simulink model "VACModel"  (Simulink 8.3)
settings: Solver=ode1  SolverMode=MultiTasking  StartTime=0.0  StopTime=24  FixedStep=Ts_base  MaxStep=Ts_base  MinStep=1e-6  RelTol=1e-6
PreLoadFcn:
  | initModel
StopFcn:
  | overview
undefined symbols (not defined in the file): automatic, controller_sampling_frequency, Fixed, gcr, MVs, PI, signal, transmitter_deadtime, transmitter_sampling_frequency, Ts_save, y_ss
libraries: VAlib x96
(part 1 of 18)
settings Model: Creator=pydipalli  LastModifiedBy=lexx
settings SolverCC: AutoInsertRateTranBlk=on
settings DataIOCC: LimitDataPoints=off  SignalLoggingSaveFormat=Dataset  SaveOutput=off  SignalLogging=off  DSMLogging=off  SaveTime=off  StateSaveName=xx  TimeSaveName=tt
settings OptimizationCC: ExpressionDepthLimit=2147483647  InitFltsAndDblsToZero=on
settings DebuggingCC: AlgebraicLoopMsg=none  SaveWithDisabledLinksMsg=none  SaveWithParameterizedLinksMsg=none  SignalResolutionControl=TryResolveAllWithWarning  SolverPrmCheckMsg=none  InheritedTsInSrcMsg=none  MultiTaskDSMMsg=warning  MultiTaskCondExecSysMsg=none  FcnCallInpInsideContextMsg=UseLocalSettings  UnconnectedInputMsg=none  UnconnectedOutputMsg=none
settings HardwareCC: TargetUnknown=on
settings RTWCC: IncludeERTFirstTime=on
settings GRTTargetCC: TargetFcnLib=ansi_tfl_tmw.mat

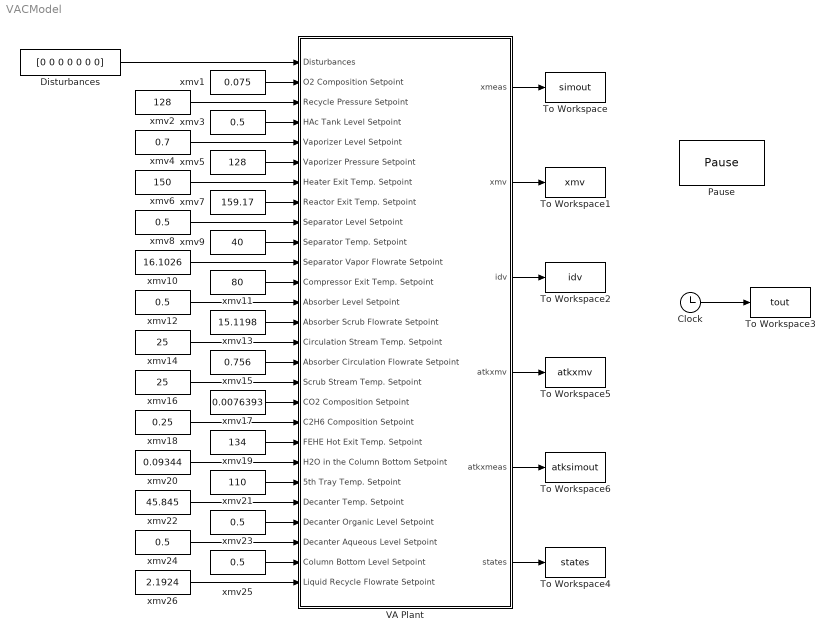
== system VACModel ==
  Clock : Clock
  Disturbances : Constant  Value=[0 0 0 0 0 0 0]
  Pause : VAlib/Pause  Value=-1
  To Workspace : ToWorkspace  VariableName=simout  SampleTime=Ts_save
  To Workspace1 : ToWorkspace  VariableName=xmv  SampleTime=Ts_save
  To Workspace2 : ToWorkspace  VariableName=idv  SampleTime=Ts_save
  To Workspace3 : ToWorkspace  VariableName=tout  SampleTime=Ts_save
      settings: Save2DSignal=2-D array (concatenate along first dimension)
  To Workspace4 : ToWorkspace  VariableName=states  SampleTime=Ts_save
  To Workspace5 : ToWorkspace  VariableName=atkxmv  SampleTime=Ts_save
  To Workspace6 : ToWorkspace  VariableName=atksimout  SampleTime=Ts_save
  VA Plant : Subsystem
  xmv1 : Constant  Value=0.075
  xmv10 : Constant  Value=16.1026
  xmv11 : Constant  Value=80
  xmv{3,8,12,23..25} (6 alike) : Constant  Value=0.5
  xmv13 : Constant  Value=15.1198
  xmv14 : Constant  Value=25
  xmv15 : Constant  Value=0.756
  xmv16 : Constant  Value=25
  xmv17 : Constant  Value=0.0076393
  xmv18 : Constant  Value=0.25
  xmv19 : Constant  Value=134
  xmv2 : Constant  Value=128
  xmv20 : Constant  Value=0.09344
  xmv21 : Constant  Value=110
  xmv22 : Constant  Value=45.845
  xmv26 : Constant  Value=2.1924
  xmv4 : Constant  Value=0.7
  xmv5 : Constant  Value=128
  xmv6 : Constant  Value=150
  xmv7 : Constant  Value=159.17
  xmv9 : Constant  Value=40
  wires:
  VA Plant/1(xmeas) -> To Workspace/1
  xmv2/1 -> VA Plant/3(Recycle Pressure Setpoint)
  VA Plant/2(xmv) -> To Workspace1/1
  VA Plant/3(idv) -> To Workspace2/1
  Clock/1 -> To Workspace3/1
  Disturbances/1 -> VA Plant/1(Disturbances)
  VA Plant/4(atkxmv) -> To Workspace5/1
  VA Plant/5(atkxmeas) -> To Workspace6/1
  xmv1/1 -> VA Plant/2(O2 Composition Setpoint)
  xmv3/1 -> VA Plant/4(HAc Tank Level Setpoint)
  xmv4/1 -> VA Plant/5(Vaporizer Level Setpoint)
  xmv5/1 -> VA Plant/6(Vaporizer Pressure Setpoint)
  xmv6/1 -> VA Plant/7(Heater Exit Temp. Setpoint)
  xmv7/1 -> VA Plant/8(Reactor Exit Temp. Setpoint)
  xmv8/1 -> VA Plant/9(Separator Level Setpoint)
  xmv9/1 -> VA Plant/10(Separator Temp. Setpoint)
  xmv10/1 -> VA Plant/11(Separator Vapor Flowrate Setpoint)
  xmv11/1 -> VA Plant/12(Compressor Exit Temp. Setpoint)
  xmv12/1 -> VA Plant/13(Absorber Level Setpoint)
  xmv13/1 -> VA Plant/14(Absorber Scrub Flowrate Setpoint)
  xmv14/1 -> VA Plant/15(Circulation Stream Temp. Setpoint)
  xmv15/1 -> VA Plant/16(Absorber Circulation Flowrate Setpoint)
  xmv16/1 -> VA Plant/17(Scrub Stream Temp. Setpoint)
  xmv17/1 -> VA Plant/18(CO2 Composition Setpoint)
  xmv18/1 -> VA Plant/19(C2H6 Composition Setpoint)
  xmv19/1 -> VA Plant/20(FEHE Hot Exit Temp. Setpoint)
  xmv20/1 -> VA Plant/21(H2O in the Column Bottom Setpoint)
  xmv21/1 -> VA Plant/22(5th Tray Temp. Setpoint)
  xmv22/1 -> VA Plant/23(Decanter Temp. Setpoint)
  xmv23/1 -> VA Plant/24(Decanter Organic Level Setpoint)
  xmv24/1 -> VA Plant/25(Decanter Aqueous Level Setpoint)
  xmv25/1 -> VA Plant/26(Column Bottom Level Setpoint)
  xmv26/1 -> VA Plant/27(Liquid Recycle Flowrate Setpoint)
  VA Plant/6(states) -> To Workspace4/1

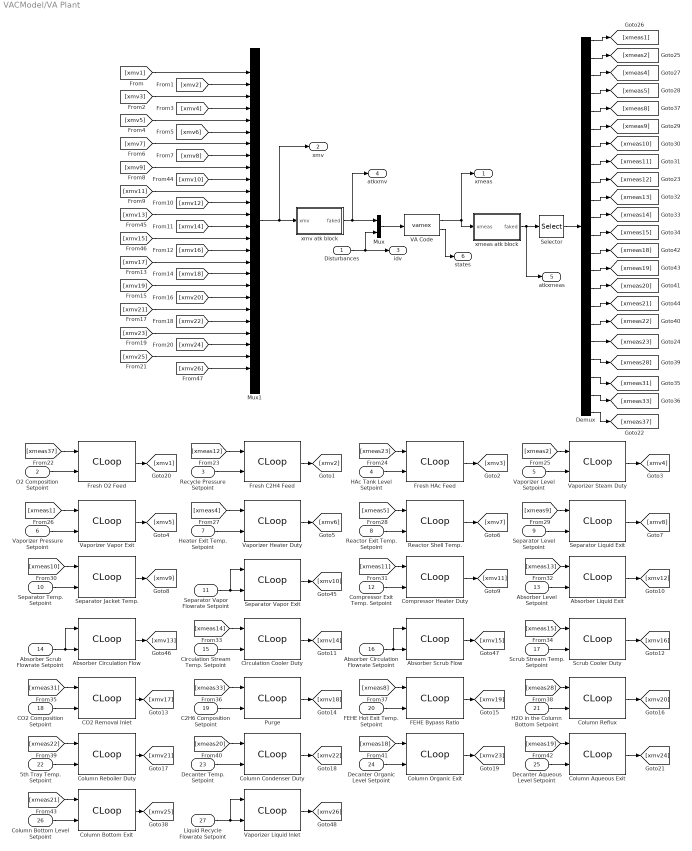
== system VACModel/VA Plant ==
  Disturbances : Inport
  O2 Composition Setpoint : Inport  Port=2
  Recycle Pressure Setpoint : Inport  Port=3
  HAc Tank Level Setpoint : Inport  Port=4
  Vaporizer Level Setpoint : Inport  Port=5
  Vaporizer Pressure Setpoint : Inport  Port=6
  Heater Exit Temp. Setpoint : Inport  Port=7
  Reactor Exit Temp. Setpoint : Inport  Port=8
  Separator Level Setpoint : Inport  Port=9
  Separator Temp. Setpoint : Inport  Port=10
  Separator Vapor Flowrate Setpoint : Inport  Port=11
  Compressor Exit Temp. Setpoint : Inport  Port=12
  Absorber Level Setpoint : Inport  Port=13
  Absorber Scrub Flowrate Setpoint : Inport  Port=14
  Circulation Stream Temp. Setpoint : Inport  Port=15
  Absorber Circulation Flowrate Setpoint : Inport  Port=16
  Scrub Stream Temp. Setpoint : Inport  Port=17
  CO2 Composition Setpoint : Inport  Port=18
  C2H6 Composition Setpoint : Inport  Port=19
  FEHE Hot Exit Temp. Setpoint : Inport  Port=20
  H2O in the Column Bottom Setpoint : Inport  Port=21
  5th Tray Temp. Setpoint : Inport  Port=22
  Decanter Temp. Setpoint : Inport  Port=23
  Decanter Organic Level Setpoint : Inport  Port=24
  Decanter Aqueous Level Setpoint : Inport  Port=25
  Column Bottom Level Setpoint : Inport  Port=26
  Liquid Recycle Flowrate Setpoint : Inport  Port=27
  Absorber Circulation Flow : VAlib/CLoop  ctype=2 (Fixed)  mode=1 (automatic)  gain=0  reset=0  csampling=controller_sampling_frequency(13)  lowmeas=0  highmeas=100  lowmv=0  highmv=50  deadtime=transmitter_deadtime(13)  tau=transmitter_lag  tsampling=transmitter_sampling_frequency(13)  x0mv=MVs(13)  x0xs=y_ss(13)  x0sp=str2num(get_param([gcr '/xmv13'], 'Value'))
  Absorber Liquid Exit : VAlib/CLoop  ctype=1 (Proportional only)  mode=1 (automatic)  gain=-5  reset=100  csampling=controller_sampling_frequency(12)  lowmeas=0  highmeas=1  lowmv=0  highmv=4.536  deadtime=transmitter_deadtime(12)  tau=transmitter_lag  tsampling=transmitter_sampling_frequency(12)  x0mv=MVs(12)  x0xs=y_ss(13)  x0sp=str2num(get_param([gcr '/xmv12'], 'Value'))
  Absorber Scrub Flow : VAlib/CLoop  ctype=2 (Fixed)  mode=1 (automatic)  gain=0  reset=0  csampling=controller_sampling_frequency(15)  lowmeas=0  highmeas=100  lowmv=0  highmv=7.560  deadtime=transmitter_deadtime(15)  tau=transmitter_lag  tsampling=transmitter_sampling_frequency(15)  x0mv=MVs(15)  x0xs=y_ss(15)  x0sp=str2num(get_param([gcr '/xmv15'], 'Value'))
  CO2 Removal Inlet : VAlib/CLoop  ctype=1 (Proportional only)  mode=1 (automatic)  gain=-1  reset=100  csampling=controller_sampling_frequency(17)  lowmeas=0  highmeas=0.5  lowmv=0  highmv=22.68  deadtime=transmitter_deadtime(17)  tau=transmitter_lag  tsampling=transmitter_sampling_frequency(17)  x0mv=MVs(17)  x0xs=y_ss(31)  x0sp=str2num(get_param([gcr '/xmv17'], 'Value'))
  Circulation Cooler Duty : VAlib/CLoop  ctype=0 (PI)  mode=1 (automatic)  gain=-1  reset=5  csampling=controller_sampling_frequency(14)  lowmeas=10  highmeas=40  lowmv=0  highmv=30000  deadtime=transmitter_deadtime(14)  tau=transmitter_lag  tsampling=transmitter_sampling_frequency(14)  x0mv=MVs(14)  x0xs=y_ss(14)  x0sp=str2num(get_param([gcr '/xmv14'], 'Value'))
  Column Aqueous Exit : VAlib/CLoop  ctype=1 (Proportional only)  mode=1 (automatic)  gain=-1  reset=100  csampling=controller_sampling_frequency(24)  lowmeas=0  highmeas=1  lowmv=0  highmv=2.4  deadtime=transmitter_deadtime(24)  tau=transmitter_lag  tsampling=transmitter_sampling_frequency(24)  x0mv=MVs(24)  x0xs=y_ss(19)  x0sp=str2num(get_param([gcr '/xmv24'], 'Value'))
  Column Bottom Exit : VAlib/CLoop  ctype=1 (Proportional only)  mode=1 (automatic)  gain=-1  reset=100  csampling=controller_sampling_frequency(25)  lowmeas=0  highmeas=1  lowmv=0  highmv=4.536  deadtime=transmitter_deadtime(25)  tau=transmitter_lag  tsampling=transmitter_sampling_frequency(25)  x0mv=MVs(25)  x0xs=y_ss(21)  x0sp=str2num(get_param([gcr '/xmv25'], 'Value'))
  Column Condenser Duty : VAlib/CLoop  ctype=0 (PI)  mode=1 (automatic)  gain=-1  reset=5  csampling=controller_sampling_frequency(22)  lowmeas=40  highmeas=50  lowmv=0  highmv=150000  deadtime=transmitter_deadtime(22)  tau=transmitter_lag  tsampling=transmitter_sampling_frequency(22)  x0mv=MVs(22)  x0xs=y_ss(20)  x0sp=str2num(get_param([gcr '/xmv22'], 'Value'))
  Column Organic Exit : VAlib/CLoop  ctype=1 (Proportional only)  mode=1 (automatic)  gain=-1  reset=100  csampling=controller_sampling_frequency(23)  lowmeas=0  highmeas=1  lowmv=0  highmv=2.4  deadtime=transmitter_deadtime(23)  tau=transmitter_lag  tsampling=transmitter_sampling_frequency(23)  x0mv=MVs(23)  x0xs=y_ss(18)  x0sp=str2num(get_param([gcr '/xmv23'], 'Value'))
  Column Reboiler Duty : VAlib/CLoop  ctype=0 (PI)  mode=1 (automatic)  gain=20  reset=30  csampling=controller_sampling_frequency(21)  lowmeas=0  highmeas=120  lowmv=0  highmv=100000  deadtime=transmitter_deadtime(21)  tau=transmitter_lag  tsampling=transmitter_sampling_frequency(21)  x0mv=MVs(21)  x0xs=y_ss(22)  x0sp=str2num(get_param([gcr '/xmv21'], 'Value'))
  Column Reflux : VAlib/CLoop  ctype=0 (PI)  mode=1 (automatic)  gain=-0.5  reset=60  csampling=controller_sampling_frequency(20)  lowmeas=0  highmeas=0.2  lowmv=0  highmv=7.56  deadtime=transmitter_deadtime(20)  tau=transmitter_lag  tsampling=transmitter_sampling_frequency(20)  x0mv=MVs(20)  x0xs=y_ss(28)  x0sp=str2num(get_param([gcr '/xmv20'], 'Value'))
  Compressor Heater Duty : VAlib/CLoop  ctype=0 (PI)  mode=1 (automatic)  gain=-1  reset=5  csampling=controller_sampling_frequency(11)  lowmeas=70  highmeas=90  lowmv=0  highmv=50000  deadtime=transmitter_deadtime(11)  tau=transmitter_lag  tsampling=transmitter_sampling_frequency(11)  x0mv=MVs(11)  x0xs=y_ss(11)  x0sp=str2num(get_param([gcr '/xmv11'], 'Value'))
  Demux : Demux  Outputs=22
  FEHE Bypass Ratio : VAlib/CLoop  ctype=0 (PI)  mode=1 (automatic)  gain=5  reset=10  csampling=controller_sampling_frequency(19)  lowmeas=0  highmeas=200  lowmv=0  highmv=1  deadtime=transmitter_deadtime(19)  tau=transmitter_lag  tsampling=transmitter_sampling_frequency(19)  x0mv=MVs(19)  x0xs=y_ss(8)  x0sp=str2num(get_param([gcr '/xmv19'], 'Value'))
  Fresh C2H4 Feed : VAlib/CLoop  ctype=0 (PI)  mode=1 (automatic)  gain=0.3  reset=20  csampling=controller_sampling_frequency(2)  lowmeas=0  highmeas=200  lowmv=0  highmv=7.56  deadtime=transmitter_deadtime(2)  tau=transmitter_lag  tsampling=transmitter_sampling_frequency(2)  x0mv=MVs(2)  x0xs=y_ss(12)  x0sp=str2num(get_param([gcr '/xmv2'], 'Value'))
  Fresh HAc Feed : VAlib/CLoop  ctype=1 (Proportional only)  mode=1 (automatic)  gain=2  reset=100  csampling=controller_sampling_frequency(3)  lowmeas=0  highmeas=1  lowmv=0  highmv=4.536  deadtime=transmitter_deadtime(3)  tau=transmitter_lag  tsampling=transmitter_sampling_frequency(3)  x0mv=MVs(3)  x0xs=y_ss(23)  x0sp=str2num(get_param([gcr '/xmv3'], 'Value'))
  Fresh O2 Feed : VAlib/CLoop  ctype=0 (PI)  mode=1 (automatic)  gain=5  reset=10  csampling=controller_sampling_frequency(1)  lowmeas=0  highmeas=0.2  lowmv=0  highmv=2.268  deadtime=transmitter_deadtime(1)  tau=transmitter_lag  tsampling=transmitter_sampling_frequency(1)  x0mv=MVs(1)  x0xs=y_ss(37)  x0sp=str2num(get_param([gcr '/xmv1'], 'Value'))
  Mux : Mux  Inputs=2
  Mux1 : Mux  Inputs=26
  Purge : VAlib/CLoop  ctype=1 (Proportional only)  mode=1 (automatic)  gain=-1  reset=100  csampling=controller_sampling_frequency(18)  lowmeas=0  highmeas=1  lowmv=0  highmv=0.02268  deadtime=transmitter_deadtime(18)  tau=transmitter_lag  tsampling=transmitter_sampling_frequency(18)  x0mv=MVs(18)  x0xs=y_ss(33)  x0sp=str2num(get_param([gcr '/xmv18'], 'Value'))
  Reactor Shell Temp. : VAlib/CLoop  ctype=0 (PI)  mode=1 (automatic)  gain=3  reset=10  csampling=controller_sampling_frequency(7)  lowmeas=0  highmeas=200  lowmv=110  highmv=150  deadtime=transmitter_deadtime(7)  tau=transmitter_lag  tsampling=transmitter_sampling_frequency(7)  x0mv=MVs(7)  x0xs=y_ss(5)  x0sp=str2num(get_param([gcr '/xmv7'], 'Value'))
  Scrub Cooler Duty : VAlib/CLoop  ctype=0 (PI)  mode=1 (automatic)  gain=-1  reset=5  csampling=controller_sampling_frequency(16)  lowmeas=10  highmeas=40  lowmv=0  highmv=5000  deadtime=transmitter_deadtime(16)  tau=transmitter_lag  tsampling=transmitter_sampling_frequency(16)  x0mv=MVs(16)  x0xs=y_ss(15)  x0sp=str2num(get_param([gcr '/xmv16'], 'Value'))
  Selector : Selector  InputPortWidth=43  Indices=[1,2,4,5,8,9,10,11,12,13,14,15,18,19,20,21,22,23,28,31,33,37]
  Separator Jacket Temp. : VAlib/CLoop  ctype=0 (PI)  mode=1 (automatic)  gain=-5  reset=20  csampling=controller_sampling_frequency(9)  lowmeas=0  highmeas=80  lowmv=0  highmv=80  deadtime=transmitter_deadtime(9)  tau=transmitter_lag  tsampling=transmitter_sampling_frequency(9)  x0mv=MVs(9)  x0xs=y_ss(10)  x0sp=str2num(get_param([gcr '/xmv9'], 'Value'))
  Separator Liquid Exit : VAlib/CLoop  ctype=1 (Proportional only)  mode=1 (automatic)  gain=-5  reset=100  csampling=controller_sampling_frequency(8)  lowmeas=0  highmeas=1  lowmv=0  highmv=4.536  deadtime=transmitter_deadtime(8)  tau=transmitter_lag  tsampling=transmitter_sampling_frequency(8)  x0mv=MVs(8)  x0xs=y_ss(9)  x0sp=str2num(get_param([gcr '/xmv8'], 'Value'))
  Separator Vapor Exit : VAlib/CLoop  ctype=2 (Fixed)  mode=1 (automatic)  gain=0  reset=0  csampling=controller_sampling_frequency(10)  lowmeas=0  highmeas=100  lowmv=0  highmv=30  deadtime=transmitter_deadtime(10)  tau=transmitter_lag  tsampling=transmitter_sampling_frequency(10)  x0mv=MVs(10)  x0xs=y_ss(10)  x0sp=str2num(get_param([gcr '/xmv10'], 'Value'))
  VA Code : S-Function  FunctionName=vamex  Parameters=[]  EnableBusSupport=off
  Vaporizer Heater Duty : VAlib/CLoop  ctype=0 (PI)  mode=1 (automatic)  gain=1  reset=5  csampling=controller_sampling_frequency(6)  lowmeas=120  highmeas=170  lowmv=0  highmv=15000  deadtime=transmitter_deadtime(6)  tau=transmitter_lag  tsampling=transmitter_sampling_frequency(6)  x0mv=MVs(6)  x0xs=y_ss(4)  x0sp=str2num(get_param([gcr '/xmv6'], 'Value'))
  Vaporizer Liquid Inlet : VAlib/CLoop  ctype=2 (Fixed)  mode=1 (automatic)  gain=0  reset=0  csampling=controller_sampling_frequency(26)  lowmeas=0  highmeas=100  lowmv=0  highmv=4.536  deadtime=transmitter_deadtime(26)  tau=transmitter_lag  tsampling=transmitter_sampling_frequency(26)  x0mv=MVs(26)  x0xs=y_ss(26)  x0sp=str2num(get_param([gcr '/xmv26'], 'Value'))
  Vaporizer Steam Duty : VAlib/CLoop  ctype=0 (PI)  mode=1 (automatic)  gain=-0.1  reset=30  csampling=controller_sampling_frequency(4)  lowmeas=0  highmeas=1  lowmv=0  highmv=1433400  deadtime=transmitter_deadtime(4)  tau=transmitter_lag  tsampling=transmitter_sampling_frequency(4)  x0mv=MVs(4)  x0xs=y_ss(2)  x0sp=str2num(get_param([gcr '/xmv4'], 'Value'))
  Vaporizer Vapor Exit : VAlib/CLoop  ctype=0 (PI)  mode=1 (automatic)  gain=-5  reset=10  csampling=controller_sampling_frequency(5)  lowmeas=0  highmeas=200  lowmv=0  highmv=50  deadtime=transmitter_deadtime(5)  tau=transmitter_lag  tsampling=transmitter_sampling_frequency(5)  x0mv=MVs(5)  x0xs=y_ss(1)  x0sp=str2num(get_param([gcr '/xmv5'], 'Value'))
  xmeas atk block : Subsystem
  xmv atk block : Subsystem
  xmeas : Outport
  xmv : Outport  Port=2
  idv : Outport  Port=3
  atkxmv : Outport  Port=4
  atkxmeas : Outport  Port=5
  states : Outport  Port=6
  wires:
  Mux/1 -> VA Code/1
  Disturbances/1 -> Mux/2, idv/1
  VA Code/1 -> xmeas atk block/1(xmeas), xmeas/1
  [xmv1] -> Mux1/1
  [xmv2] -> Mux1/2
  [xmv3] -> Mux1/3
  [xmv4] -> Mux1/4
  [xmv6] -> Mux1/6
  [xmv7] -> Mux1/7
  [xmv8] -> Mux1/8
  Mux1/1 -> xmv/1, xmv atk block/1(xmv)
  xmv atk block/1(faked) -> atkxmv/1, Mux/1
  xmeas atk block/1(faked) -> Selector/1, atkxmeas/1
  Selector/1 -> Demux/1
  [xmv5] -> Mux1/5
  [xmv9] -> Mux1/9
  [xmv11] -> Mux1/11
  [xmv12] -> Mux1/12
  [xmv14] -> Mux1/14
  [xmv16] -> Mux1/16
  [xmv17] -> Mux1/17
  [xmv18] -> Mux1/18
  [xmv19] -> Mux1/19
  [xmv20] -> Mux1/20
  [xmv21] -> Mux1/21
  [xmv22] -> Mux1/22
  [xmv23] -> Mux1/23
  [xmv24] -> Mux1/24
  [xmv25] -> Mux1/25
  Demux/2 -> [xmeas2]
  Demux/1 -> [xmeas1]
  Demux/3 -> [xmeas4]
  Demux/4 -> [xmeas5]
  Demux/12 -> [xmeas15]
  Demux/11 -> [xmeas14]
  Demux/10 -> [xmeas13]
  Demux/9 -> [xmeas12]
  Demux/8 -> [xmeas11]
  Demux/7 -> [xmeas10]
  Demux/6 -> [xmeas9]
  Demux/5 -> [xmeas8]
  Demux/13 -> [xmeas18]
  Demux/14 -> [xmeas19]
  Demux/15 -> [xmeas20]
  Demux/16 -> [xmeas21]
  Demux/17 -> [xmeas22]
  Demux/18 -> [xmeas23]
  Demux/19 -> [xmeas28]
  Demux/20 -> [xmeas31]
  Demux/21 -> [xmeas33]
  Demux/22 -> [xmeas37]
  [xmeas37] -> Fresh O2 Feed/1
  O2 Composition Setpoint/1 -> Fresh O2 Feed/2
  [xmeas13] -> Absorber Liquid Exit/1
  Absorber Level Setpoint/1 -> Absorber Liquid Exit/2
  Absorber Liquid Exit/1 -> [xmv12]
  [xmeas12] -> Fresh C2H4 Feed/1
  Recycle Pressure Setpoint/1 -> Fresh C2H4 Feed/2
  [xmeas23] -> Fresh HAc Feed/1
  HAc Tank Level Setpoint/1 -> Fresh HAc Feed/2
  [xmeas2] -> Vaporizer Steam Duty/1
  Vaporizer Level Setpoint/1 -> Vaporizer Steam Duty/2
  [xmeas4] -> Vaporizer Heater Duty/1
  Heater Exit Temp. Setpoint/1 -> Vaporizer Heater Duty/2
  [xmeas5] -> Reactor Shell Temp./1
  Reactor Exit Temp. Setpoint/1 -> Reactor Shell Temp./2
  Reactor Shell Temp./1 -> [xmv7]
  [xmeas9] -> Separator Liquid Exit/1
  Separator Liquid Exit/1 -> [xmv8]
  Separator Level Setpoint/1 -> Separator Liquid Exit/2
  [xmeas10] -> Separator Jacket Temp./1
  Separator Temp. Setpoint/1 -> Separator Jacket Temp./2
  Separator Jacket Temp./1 -> [xmv9]
  [xmeas11] -> Compressor Heater Duty/1
  Compressor Exit Temp. Setpoint/1 -> Compressor Heater Duty/2
  Compressor Heater Duty/1 -> [xmv11]
  [xmeas14] -> Circulation Cooler Duty/1
  Circulation Cooler Duty/1 -> [xmv14]
  Circulation Stream Temp. Setpoint/1 -> Circulation Cooler Duty/2
  [xmeas15] -> Scrub Cooler Duty/1
  Scrub Stream Temp. Setpoint/1 -> Scrub Cooler Duty/2
  Scrub Cooler Duty/1 -> [xmv16]
  [xmeas31] -> CO2 Removal Inlet/1
  CO2 Removal Inlet/1 -> [xmv17]
  CO2 Composition Setpoint/1 -> CO2 Removal Inlet/2
  [xmeas33] -> Purge/1
  Purge/1 -> [xmv18]
  C2H6 Composition Setpoint/1 -> Purge/2
  [xmeas8] -> FEHE Bypass Ratio/1
  FEHE Hot Exit Temp. Setpoint/1 -> FEHE Bypass Ratio/2
  FEHE Bypass Ratio/1 -> [xmv19]
  [xmeas28] -> Column Reflux/1
  H2O in the Column Bottom Setpoint/1 -> Column Reflux/2
  Column Reflux/1 -> [xmv20]
  [xmeas22] -> Column Reboiler Duty/1
  5th Tray Temp. Setpoint/1 -> Column Reboiler Duty/2
  Column Reboiler Duty/1 -> [xmv21]
  [xmeas20] -> Column Condenser Duty/1
  Decanter Temp. Setpoint/1 -> Column Condenser Duty/2
  Column Condenser Duty/1 -> [xmv22]
  [xmeas18] -> Column Organic Exit/1
  Column Organic Exit/1 -> [xmv23]
  Decanter Organic Level Setpoint/1 -> Column Organic Exit/2
  [xmeas19] -> Column Aqueous Exit/1
  Decanter Aqueous Level Setpoint/1 -> Column Aqueous Exit/2
  Column Aqueous Exit/1 -> [xmv24]
  [xmeas21] -> Column Bottom Exit/1
  Column Bottom Level Setpoint/1 -> Column Bottom Exit/2
  Column Bottom Exit/1 -> [xmv25]
  VA Code/2 -> states/1
  Fresh O2 Feed/1 -> [xmv1]
  Fresh C2H4 Feed/1 -> [xmv2]
  Fresh HAc Feed/1 -> [xmv3]
  Vaporizer Steam Duty/1 -> [xmv4]
  Vaporizer Heater Duty/1 -> [xmv6]
  [xmeas1] -> Vaporizer Vapor Exit/1
  Vaporizer Pressure Setpoint/1 -> Vaporizer Vapor Exit/2
  Vaporizer Vapor Exit/1 -> [xmv5]
  Separator Vapor Exit/1 -> [xmv10]
  Separator Vapor Flowrate Setpoint/1 -> Separator Vapor Exit/1, Separator Vapor Exit/2
  [xmv10] -> Mux1/10
  Absorber Circulation Flow/1 -> [xmv13]
  Absorber Scrub Flowrate Setpoint/1 -> Absorber Circulation Flow/1, Absorber Circulation Flow/2
  [xmv13] -> Mux1/13
  Absorber Scrub Flow/1 -> [xmv15]
  Absorber Circulation Flowrate Setpoint/1 -> Absorber Scrub Flow/1, Absorber Scrub Flow/2
  [xmv15] -> Mux1/15
  Vaporizer Liquid Inlet/1 -> [xmv26]
  Liquid Recycle Flowrate Setpoint/1 -> Vaporizer Liquid Inlet/1, Vaporizer Liquid Inlet/2
  [xmv26] -> Mux1/26
